simulink model "expt_6_c"  (R2018b)
settings: Solver=VariableStepAuto  StartTime=0.0  StopTime=0.1  RelTol=1e-3
libraries: dspquant2 x1, commutil2 x1, dspsigops x1
settings Model: Creator=sangh  LastModifiedBy=sangh

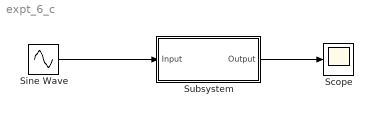
== system expt_6_c ==
  Scope : Scope
  Sine Wave : Sin  Frequency=2*pi*500  SampleTime=2e-6
  Subsystem : Subsystem
  wires:
  Sine Wave/1 -> Subsystem/1(Input)
  Subsystem/1(Output) -> Scope/1

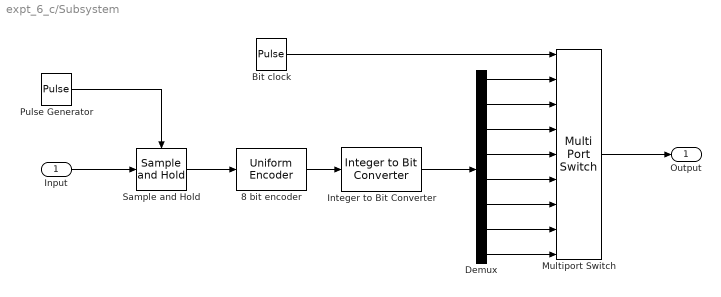
== system expt_6_c/Subsystem ==
  Input : Inport
  8 bit encoder : dspquant2/Uniform Encoder  peak=1  bits=8  otype=Unsigned integer
      settings: SourceProductName=DSP System Toolbox
  Bit clock : DiscretePulseGenerator  PulseType=Time based  Period=1/50e3  PulseWidth=50
  Demux : Demux  Outputs=8
  Integer to Bit Converter : commutil2/Integer to Bit Converter  nbits=8  signedInputValues=Signed  bitOrder=MSB first  outDtype=Inherit via internal rule
  Multiport Switch : MultiPortSwitch  Inputs=8  DiagnosticForDefault=Warning  SaturateOnIntegerOverflow=on  InputSameDT=on
  Pulse Generator : DiscretePulseGenerator  PulseType=Time based  Period=1/20e3  PulseWidth=10
  Sample and Hold : dspsigops/Sample and Hold  trig=Rising edge  initCond=0  latchinput=off
  Output : Outport
  wires:
  Input/1 -> Sample and Hold/1
  Pulse Generator/1 -> Sample and Hold/Trigger
  Sample and Hold/1 -> 8 bit encoder/1
  8 bit encoder/1 -> Integer to Bit Converter/1
  Integer to Bit Converter/1 -> Demux/1
  Demux/1 -> Multiport Switch/2
  Demux/2 -> Multiport Switch/3
  Demux/3 -> Multiport Switch/4
  Demux/4 -> Multiport Switch/5
  Demux/5 -> Multiport Switch/6
  Demux/6 -> Multiport Switch/7
  Demux/7 -> Multiport Switch/8
  Demux/8 -> Multiport Switch/9
  Bit clock/1 -> Multiport Switch/1
  Multiport Switch/1 -> Output/1
